simulink model "WL_main_simulink"  (R2025a)
settings: Solver=ode4  StartTime=0.0  StopTime=T_sim  FixedStep=Dt_sim  RelTol=1e-3
InitFcn:
  | % --- AUTOMATIC WINGLOOP PYTHON SERVER STARTUP ---
  | fprintf('[Simulink] Preparing WingLoop simulation...\n');
  | 
  | gust_choice = questdlg('Do you want to include the gust file (gust_H40.gust)?', ...
  |     'Gust Configuration', 'Yes', 'No', 'No');
  | if isempty(gust_choice)
  |     gust_choice = 'No';
  | end
  | 
  | video_choice = questdlg('Do you want to generate a video after the simulation?', ...
  |     'Video Configuration', 'Yes', 'No', 'No');
  | if isempty(video_choice)
  |     video_choice = 'No';
  | end
  | 
  | model_file = get_param(bdroot, 'FileName');
  | simulink_controller_dir = fileparts(model_file);
  | wingloop_testrun_dir_win = fileparts(simulink_controller_dir);
  | 
  | wingloop_testrun_dir_wsl = strrep(wingloop_testrun_dir_win, '\\wsl.localhost\ubuntu', '');
  | wingloop_testrun_dir_wsl = strrep(wingloop_testrun_dir_wsl, '\', '/');
  | 
  | fprintf('[Simulink] WingLoop Windows directory:\n%s\n', wingloop_testrun_dir_win);
  | fprintf('[Simulink] WingLoop WSL directory:\n%s\n', wingloop_testrun_dir_wsl);
  | 
  | file_inputs = fullfile(wingloop_testrun_dir_win, 'python_inputs.txt');
  | 
  | fid = fopen(file_inputs, 'w');
  | 
  | if fid < 0
  |     error('[Simulink] Unable to create python_inputs.txt at:\n%s', file_inputs);
  | end
  | 
  | fprintf(fid, '1\n');
  | 
  | if strcmp(gust_choice, 'Yes')
  |     fprintf(fid, 'y\n');
  | else
  |     fprintf(fid, 'n\n');
  | end
  | 
  | if strcmp(video_choice, 'Yes')
  |     fprintf(fid, 'y\n');
  |     fprintf(fid, 'gif\n');
  |     fprintf(fid, 'medium\n');
  |     fprintf(fid, 'Y\n');
  | else
  |     fprintf(fid, 'n\n');
  | end
  | 
  | fclose(fid);
  | 
  | fprintf('[Simulink] Input file written to:\n%s\n', file_inputs);
  | 
  | cmd_wsl = sprintf(['start "WingLoop Python Server" wsl -e bash -ic ', ...
  |     '"source ~/miniconda3/etc/profile.d/conda.sh && ', ...
  |     'conda activate WINGLOOP && ', ...
  |     'cd %s && ', ...
  |     'echo ACTIVE_CONDA_ENV=$CONDA_DEFAULT_ENV && ', ...
  |     'which python3 && ', ...
  |     'python3 wingloop_testrun.py < python_inputs.txt; ', ...
  |     'exec bash"'], ...
  |     wingloop_testrun_dir_wsl);
  | 
  | fprintf('[Simulink] Launch command:\n%s\n', cmd_wsl);
  | system(cmd_wsl);
values from neighbouring files (symbols this model uses):
  Dt_asw = 0.1    [WL_main.m]
  u_trim = [0, F2ref, F3ref, 0, E2ref, E2ref]    [WL_main.m]
undefined symbols (not defined in the file or in its folder): FullModel
settings Model: SimulationMode=accelerator  Creator=lpmat  LastModifiedBy=lpmat

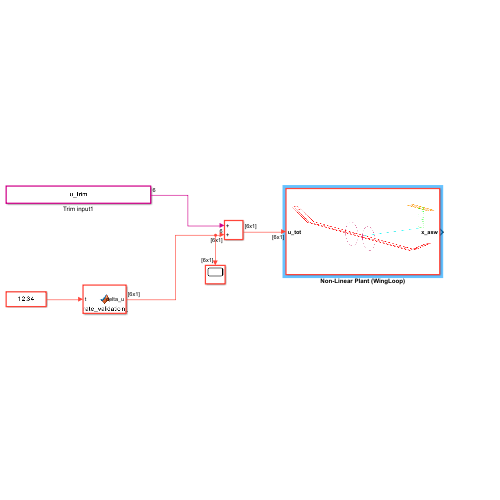
[thumbnail: Simulink's stored preview of the top-level diagram]
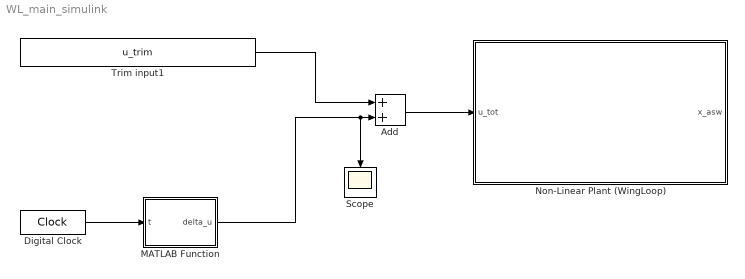
== system WL_main_simulink ==
  Add : Sum
  Digital Clock : DigitalClock  SampleTime=Dt_asw
  MATLAB Function : MATLAB Function  TreatAsAtomicUnit=on
  Non-Linear Plant (WingLoop) : Subsystem
      mask Display: image('Screenshot 2026-03-18 123158.png');
  Scope : Scope
  Trim input1 : Constant  Value=u_trim
  wires:
  Add/1 -> Non-Linear Plant (WingLoop)/1(u_tot)
  Trim input1/1 -> Add/1
  Digital Clock/1 -> MATLAB Function/1(t)
  MATLAB Function/1(delta_u) -> Scope/1, Add/2

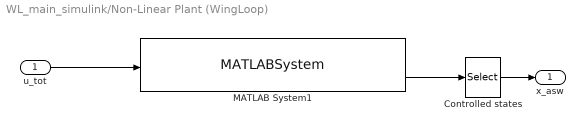
== system WL_main_simulink/Non-Linear Plant (WingLoop) ==
  u_tot : Inport
  Controlled states : Selector  InputPortWidth=1894  IndexOptions=Index vector (dialog)  Indices=[1:1882]  OutputSizes=1
  MATLAB System1 : MATLABSystem  System=AswingPlant  ServerHost=localhost  ServerPort=5005  NumModalStates=ROM.n_modal  NumPhysicalStates=FullModel.n_orig+ FullModel.n_in  SimulateUsing=Interpreted execution
      mask Type: AswingPlant
  x_asw : Outport
  wires:
  MATLAB System1/2 -> Controlled states/1
  u_tot/1 -> MATLAB System1/1
  Controlled states/1 -> x_asw/1

== matlab function WL_main_simulink/MATLAB Function ==
  data: t input; delta_u output
function delta_u = generate_validation_cmd(t)
    % Parametri della manovra
    t_start = 1.0;  % Inizio incremento a 1 secondo
    tau = 1.0;      % Costante di tempo (velocità della curva)
    
    % Inizializziamo il vettore delta_u (6 canali)
    delta_u = zeros(6, 1);
    
    if t >= t_start
        % Calcolo della dinamica esponenziale: 1 - exp(-t/tau)
        % Arriva al 99% del target in circa 5*tau secondi
        dinamica = (1.0 - exp(-(t - t_start) / tau));
        
        % Canale 2: Flap (+1 grado)
        delta_u(2) = 1.0 * dinamica;
        
        
    end
end
